simulink model "pendulum_sim"  (R2019b)
settings: Solver=VariableStepAuto  StartTime=0.0  StopTime=10  RelTol=1e-3  EnableMultiTasking=on
InitFcn:
  | addpath ./..
  | pendulumParam
undefined symbols (not defined in the file): pendulum_animation
settings Model: Creator=beard  LastModifiedBy=JoHn
settings DataIOCC: LimitDataPoints=on  SaveFormat=Array  SignalLoggingSaveFormat=ModelDataLogs  ReturnWorkspaceOutputs=off
settings OptimizationCC: ExpressionDepthLimit=2147483647  InitFltsAndDblsToZero=on  LifeSpan=inf
settings DebuggingCC: UnderspecifiedInitializationDetection=Classic  MergeDetectMultiDrivingBlocksExec=none  SolverPrmCheckMsg=warning  FcnCallInpInsideContextMsg=warning  StateNameClashWarn=warning  SFUnexpectedBacktrackingDiag=warning  SFNoUnconditionalDefaultTransitionDiag=warning  SFExecutionAtInitializationDiag=none  ArithmeticOperatorsInVariantConditions=warning
settings HardwareCC: ProdBitPerPointer=32  ProdBitPerSizeT=32  ProdBitPerPtrDiffT=32  ProdLargestAtomicFloat=None  ProdIntDivRoundTo=Undefined  ProdEndianess=Unspecified  ProdWordSize=32  ProdHWDeviceType=32-bit Generic
settings ModelReferenceCC: PropagateSignalLabelsOutOfModel=off
settings SFSimCC: SimUseLocalCustomCode=off  CustomCodeUndefinedFunction=UseInterfaceOnly
settings RTWCC: RTWUseLocalCustomCode=off
settings CodeAppCC: StateflowObjectComments=on
settings GRTTargetCC: TargetLangStandard=C89/C90 (ANSI)  GeneratePreprocessorConditionals=Disable all  CombineOutputUpdateFcns=off  GRTInterface=on
settings ConfigComp: CovMetricSettings=dw  CovHtmlReporting=on  CovSaveCumulativeToWorkspaceVar=on  CovSaveSingleToWorkspaceVar=on  CovExternalEMLEnable=off

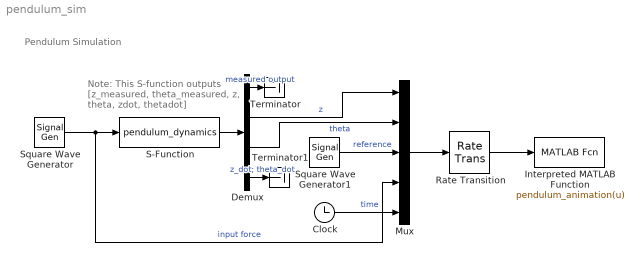
== system pendulum_sim ==
  note: Note: This S-function
      | outputs
      | [z_measured, theta_measured,
      |  z, theta, zdot, thetadot]
  note: Pendulum Simulation
  Clock : Clock
  Demux : Demux  Outputs=[2,1,1,2]
  Interpreted MATLAB Function : MATLABFcn  MATLABFcn=pendulum_animation(u)  OutputDimensions=0
  Mux : Mux  Inputs=5
  Rate Transition : RateTransition  OutPortSampleTime=P.t_plot
  S-Function : S-Function  FunctionName=pendulum_dynamics  Parameters=P  SFunctionDeploymentMode=off  EnableBusSupport=off
  Square Wave Generator : SignalGenerator  WaveForm=square  Amplitude=.2  Frequency=.5  Units=rad/sec
  Square Wave Generator1 : SignalGenerator  WaveForm=square  Units=rad/sec
  Terminator : Terminator
  Terminator1 : Terminator
  wires:
  Square Wave Generator/1 -> Mux/4, S-Function/1  "input force"
  S-Function/1 -> Demux/1
  Square Wave Generator1/1 -> Mux/3  "reference"
  Clock/1 -> Mux/5  "time"
  Mux/1 -> Rate Transition/1
  Rate Transition/1 -> Interpreted MATLAB Function/1
  Demux/4 -> Terminator1/1  "z_dot; theta_dot"
  Demux/1 -> Terminator/1  "measured output"
  Demux/2 -> Mux/1  "z"
  Demux/3 -> Mux/2  "theta"
